simulink model "MovRotSimulink"  (R2024a)
settings: Solver=ode23  StartTime=0.0  StopTime=10  RelTol=1e-3
settings Model: Creator=danid  LastModifiedBy=Hector Gael Iñiguez
settings RTWCC: GPUComputeCapability=3.5

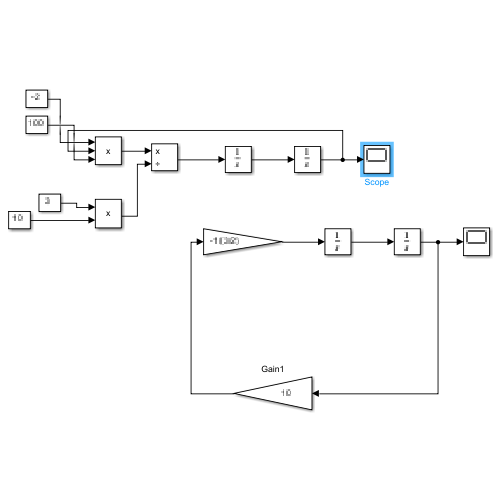
[thumbnail: Simulink's stored preview of the top-level diagram]
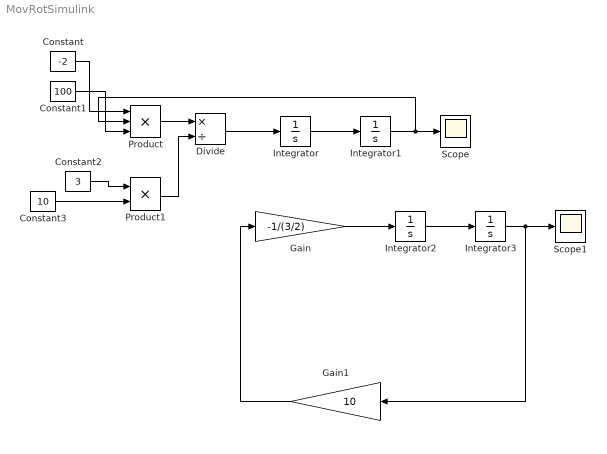
== system MovRotSimulink ==
  Constant : Constant  Value=-2
  Constant1 : Constant  Value=100
  Constant2 : Constant  Value=3
  Constant3 : Constant  Value=10
  Divide : Product  Inputs=*/
  Gain : Gain  Gain=-1/(3/2)
  Gain1 : Gain  Gain=10
  Integrator : Integrator  InitialCondition=2
  Integrator1 : Integrator
  Integrator2 : Integrator  InitialCondition=2
  Integrator3 : Integrator
  Product : Product  Inputs=3
  Product1 : Product
  Scope : Scope
  Scope1 : Scope
  wires:
  Integrator/1 -> Integrator1/1
  Integrator1/1 -> Product/2, Scope/1
  Divide/1 -> Integrator/1
  Product/1 -> Divide/1
  Product1/1 -> Divide/2
  Constant1/1 -> Product/3
  Constant2/1 -> Product1/1
  Constant3/1 -> Product1/2
  Constant/1 -> Product/1
  Integrator3/1 -> Gain1/1, Scope1/1
  Integrator2/1 -> Integrator3/1
  Gain/1 -> Integrator2/1
  Gain1/1 -> Gain/1
